simulink model "project1_Jaden"  (R2015b)
settings: Solver=ode45  SolverMode=SingleTasking  StartTime=0.0  StopTime=604800  MaxStep=1  RelTol=1e-6
undefined symbols (not defined in the file or in its folder): plecs, sigbuilder_block
settings Model: Creator=Sam Murray  LastModifiedBy=Sam Murray
settings DataIOCC: SaveFormat=Array
settings OptimizationCC: BlockReduction=off  BooleanDataType=off
settings DebuggingCC: SaveWithParameterizedLinksMsg=none  UnderspecifiedInitializationDetection=Classic  MergeDetectMultiDrivingBlocksExec=none  SignalResolutionControl=TryResolveAllWithWarning  AllowSymbolicDim=on
settings HardwareCC: ProdBitPerPointer=32  ProdLargestAtomicFloat=None  ProdIntDivRoundTo=Undefined  ProdEndianess=Unspecified  ProdWordSize=32  ProdHWDeviceType=32-bit Generic  TargetUnknown=on
settings GRTTargetCC: GeneratePreprocessorConditionals=Disable all
settings ConfigComp: CovMetricSettings=dwe  CovHtmlReporting=off  CovSaveCumulativeToWorkspaceVar=off  CovSaveSingleToWorkspaceVar=off  CovModelRefEnable=Off  CovExternalEMLEnable=on

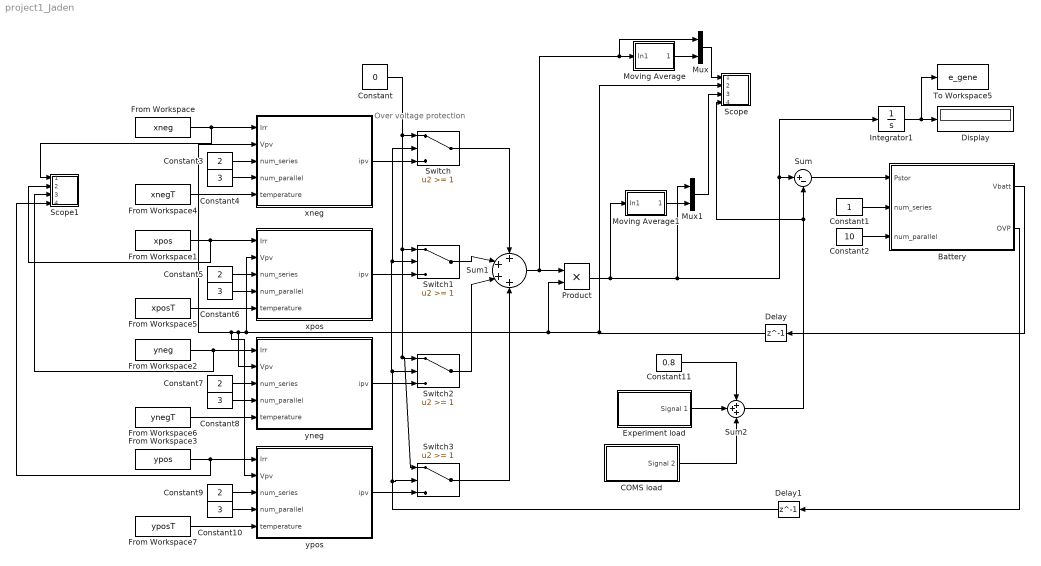
== system project1_Jaden ==
  note: Over voltage protection
  Battery : Subsystem
  COMS load : Subsystem  Tag=STV Subsys  LoadFcn=sigbuilder_block('load');  StartFcn=sigbuilder_block('start');  StopFcn=sigbuilder_block('stop');  ClipboardFcn=sigbuilder_block('clipboard');  mask(Sigbuilder block){}
      mask help: Simulink:masks:SigbuilderBlock_MD
      mask init:
      | if ~strcmp(get_param(bdroot(gcbh),'SimulationStatus'),'stopped') tuvar = sigbuilder_block('maskInit'); end
      settings: CopyFcn=sigbuilder_block('copy');  DeleteFcn=sigbuilder_block('delete');  ModelCloseFcn=sigbuilder_block('modelClose');  PreSaveFcn=sigbuilder_block('preSave');  PauseFcn=sigbuilder_block('pause');  ContinueFcn=sigbuilder_block('continue');  NameChangeFcn=sigbuilder_block('namechange');  OpenFcn=sigbuilder_block('open',[312.75 246 827.25 429 ]);  CloseFcn=sigbuilder_block('close');
      mask Display: plot(0, 0, 100, 100,[2, 2, 32, 32, 2], [68, 8, 8, 68, 68],[32, 2], [38, 38], [32, 19, 2],[53, 60, 44], [32, 17, 17, 2],[16, 16, 31, 31]);txt = getActiveGroup(gcbh);text(2, 100, txt,'verticalAlignment', 'top');
  Constant : Constant  Value=0
  Constant1 : Constant
  Constant{4,6,8,10} (4 alike) : Constant  Value=3
  Constant11 : Constant  Value=0.8
  Constant2 : Constant  Value=10
  Constant{3,5,7,9} (4 alike) : Constant  Value=2
  Delay : Delay  DelayLength=1  InitialCondition=0
  Delay1 : Delay  DelayLength=1  InitialCondition=0
  Display : Display
  Experiment load : Subsystem  Tag=STV Subsys  LoadFcn=sigbuilder_block('load');  StartFcn=sigbuilder_block('start');  StopFcn=sigbuilder_block('stop');  ClipboardFcn=sigbuilder_block('clipboard');  mask(Sigbuilder block){}
      mask help: Simulink:masks:SigbuilderBlock_MD
      mask init:
      | if ~strcmp(get_param(bdroot(gcbh),'SimulationStatus'),'stopped') tuvar = sigbuilder_block('maskInit'); end
      settings: CopyFcn=sigbuilder_block('copy');  DeleteFcn=sigbuilder_block('delete');  ModelCloseFcn=sigbuilder_block('modelClose');  PreSaveFcn=sigbuilder_block('preSave');  PauseFcn=sigbuilder_block('pause');  ContinueFcn=sigbuilder_block('continue');  NameChangeFcn=sigbuilder_block('namechange');  OpenFcn=sigbuilder_block('open',[312.75 246 827.25 429 ]);  CloseFcn=sigbuilder_block('close');
      mask Display: plot(0, 0, 100, 100,[2, 2, 32, 32, 2], [68, 8, 8, 68, 68],[32, 2], [38, 38], [32, 19, 2],[53, 60, 44], [32, 17, 17, 2],[16, 16, 31, 31]);txt = getActiveGroup(gcbh);text(2, 100, txt,'verticalAlignment', 'top');
  From Workspace : FromWorkspace  VariableName=xneg  SampleTime=0
  From Workspace1 : FromWorkspace  VariableName=xpos  SampleTime=0
  From Workspace2 : FromWorkspace  VariableName=yneg  SampleTime=0
  From Workspace3 : FromWorkspace  VariableName=ypos  SampleTime=0
  From Workspace4 : FromWorkspace  VariableName=xnegT  SampleTime=0
  From Workspace5 : FromWorkspace  VariableName=xposT  SampleTime=0
  From Workspace6 : FromWorkspace  VariableName=ynegT  SampleTime=0
  From Workspace7 : FromWorkspace  VariableName=yposT  SampleTime=0
  Integrator1 : Integrator
  Moving Average : Subsystem  Description=Replaced Block  mask(Replaced Block){}
      mask help: This block has been replaced with an empty subsystem because it used functionality that is unavailable in Simulink R2015b.
      mask Display: fprintf('Replaced: %s\n','dspstat3/Moving Average')
  Moving Average1 : Subsystem  Description=Replaced Block  mask(Replaced Block){}
      mask help: This block has been replaced with an empty subsystem because it used functionality that is unavailable in Simulink R2015b.
      mask Display: fprintf('Replaced: %s\n','dspstat3/Moving Average')
  Mux : Mux  Inputs=2
  Mux1 : Mux  Inputs=2
  Product : Product
  Scope : Subsystem  LoadFcn=plecs('sl', 300);  InitFcn=plecs('sl', 314);  StartFcn=plecs('sl', 308);  StopFcn=plecs('sl', 309);  mask{Settings=<binary blob, 1724 chars, not shown>}
      mask init:
      | plecs('sl', 315);
      settings: CopyFcn=plecs('sl', 303);  DeleteFcn=plecs('sl', 305);  UndoDeleteFcn=plecs('sl', 306);  PreSaveFcn=plecs('sl', 311);  NameChangeFcn=plecs('sl', 310);  DestroyFcn=plecs('sl', 307);  OpenFcn=plecs('sl', 302);  ErrorFcn=plerrorfcn
      mask Display: plot([0.1 0.9 0.9 0.1 0.1], [0.9 0.9 0.5 0.5 0.9])
  Scope1 : Subsystem  LoadFcn=plecs('sl', 300);  InitFcn=plecs('sl', 314);  StartFcn=plecs('sl', 308);  StopFcn=plecs('sl', 309);  mask{Settings=<binary blob, 1460 chars, not shown>}
      mask init:
      | plecs('sl', 315);
      settings: CopyFcn=plecs('sl', 303);  DeleteFcn=plecs('sl', 305);  UndoDeleteFcn=plecs('sl', 306);  PreSaveFcn=plecs('sl', 311);  NameChangeFcn=plecs('sl', 310);  DestroyFcn=plecs('sl', 307);  OpenFcn=plecs('sl', 302);  ErrorFcn=plerrorfcn
      mask Display: plot([0.1 0.9 0.9 0.1 0.1], [0.9 0.9 0.5 0.5 0.9])
  Sum : Sum  Inputs=|+-
  Sum1 : Sum  Inputs=++++
  Sum2 : Sum  Inputs=+++
  Switch{,1..3} (4 alike) : Switch  Threshold=1
  To Workspace5 : ToWorkspace  VariableName=e_gene  SaveFormat=Timeseries  SampleTime=-1
  xneg : Subsystem
  xpos : Subsystem
  yneg : Subsystem
  ypos : Subsystem
  wires:
  Constant1/1 -> Battery/2(num_series)
  Constant2/1 -> Battery/3(num_parallel)
  Constant4/1 -> xneg/4(num_parallel)
  Constant3/1 -> xneg/3(num_series)
  Sum/1 -> Battery/1(Pstor)
  From Workspace2/1 -> yneg/1(Irr), Scope1/3(3)
  From Workspace1/1 -> xpos/1(Irr), Scope1/2(2)
  From Workspace3/1 -> ypos/1(Irr), Scope1/4(4)
  Battery/1(Vbatt) -> Delay/1
  Sum1/1 -> Mux/1, Moving Average/1(In1), Product/1
  Product/1 -> Mux1/1, Integrator1/1, Sum/1, Moving Average1/1(In1)
  From Workspace/1 -> Scope1/1(1), xneg/1(Irr)
  Delay/1 -> Scope/2(2), Product/2, xpos/2(Vpv), yneg/2(Vpv), ypos/2(Vpv), xneg/2(Vpv)
  Switch/1 -> Sum1/1
  xneg/1(ipv) -> Switch/3
  Switch1/1 -> Sum1/2
  xpos/1(ipv) -> Switch1/3
  Switch2/1 -> Sum1/3
  yneg/1(ipv) -> Switch2/3
  ypos/1(ipv) -> Switch3/3
  Constant/1 -> Switch3/1, Switch2/1, Switch1/1, Switch/1
  Battery/2(OVP) -> Delay1/1
  Delay1/1 -> Switch3/2, Switch/2, Switch1/2, Switch2/2
  Integrator1/1 -> To Workspace5/1, Display/1
  Sum2/1 -> Scope/4(4), Sum/2
  Constant11/1 -> Sum2/1
  Experiment load/1(Signal 1) -> Sum2/2
  COMS load/1(Signal 2) -> Sum2/3
  Mux/1 -> Scope/1(1)
  Mux1/1 -> Scope/3(3)
  Moving Average1/1(Out1) -> Mux1/2
  Moving Average/1(Out1) -> Mux/2
  Constant5/1 -> xpos/3(num_series)
  Constant6/1 -> xpos/4(num_parallel)
  Constant7/1 -> yneg/3(num_series)
  Constant8/1 -> yneg/4(num_parallel)
  Constant9/1 -> ypos/3(num_series)
  Constant10/1 -> ypos/4(num_parallel)
  From Workspace4/1 -> xneg/5(temperature)
  From Workspace5/1 -> xpos/5(temperature)
  From Workspace6/1 -> yneg/5(temperature)
  From Workspace7/1 -> ypos/5(temperature)
  Switch3/1 -> Sum1/4

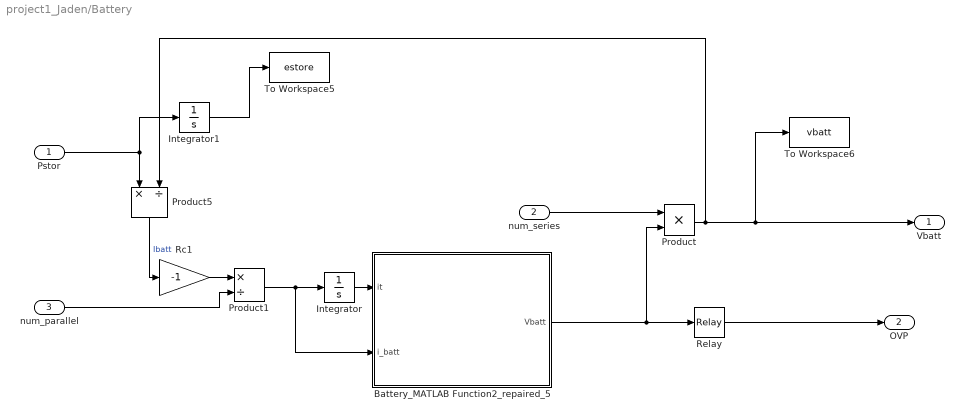
== system project1_Jaden/Battery ==
  Pstor : Inport
  num_series : Inport  Port=2
  num_parallel : Inport  Port=3
  Battery_MATLAB Function2_repaired_5 : MATLAB Function
  Integrator : Integrator  InitialCondition=4680
  Integrator1 : Integrator
  Product : Product
  Product1 : Product  Inputs=*/
  Product5 : Product  Inputs=*/  OutMin=[0]
  Rc1 : Gain  Gain=-1
  Relay : Relay  OnSwitchValue=4.2  OffSwitchValue=4.18
  To Workspace5 : ToWorkspace  VariableName=estore  SaveFormat=Timeseries  SampleTime=-1
  To Workspace6 : ToWorkspace  VariableName=vbatt  SaveFormat=Timeseries  SampleTime=-1
  Vbatt : Outport
  OVP : Outport  Port=2
  wires:
  Product/1 -> Product5/2, Vbatt/1, To Workspace6/1
  Battery_MATLAB Function2_repaired_5/1(Vbatt) -> Product/2, Relay/1
  num_series/1 -> Product/1
  num_parallel/1 -> Product1/2
  Product1/1 -> Battery_MATLAB Function2_repaired_5/2(i_batt), Integrator/1
  Integrator/1 -> Battery_MATLAB Function2_repaired_5/1(it)
  Relay/1 -> OVP/1
  Rc1/1 -> Product1/1
  Pstor/1 -> Product5/1, Integrator1/1
  Product5/1 -> Rc1/1  "Ibatt"
  Integrator1/1 -> To Workspace5/1

== system project1_Jaden/COMS load ==
  Demux : Demux  Tag=STV Demux  Outputs=1
  FromWs : FromWorkspace  Tag=STV FromWs  VariableName=tuvar  SampleTime=0
      SigBuilderData=|
      | common.afterFinalStr = 'Extrapolate'
      | common.sampleTime = 0
      | dataSet.timeRange = [0 604800]
      | dataSet.name = 'Group 1'
      | sbobj.Groups.Name = 'Group 1'
      | sbobj.Groups.Signals.Name = 'Signal 2'
      | sbobj.Groups.Signals.XData = [0 60 60 14400 14400 14460 14460 28800 28800 28860 28860 43200 43200 43260 43260 57600 57600 57660 57660 72000 72000 72060 72060 86400 86400 86460 86460 100800 100800 100860 100860 115200 115200 115260 115260 129600 129600 129660 129660 144000 144000 144060 144060 158400 158400 158460 158460 172800 172800 172860 172860 187200 187200 187260 187260 201600 201600 201660 201660 216000 216000 216060 216060 230400 230400 230460 230460 244800 244800 244860 244860 259200 259200 259260 259260 273600 273600 273660 273660 288000 288000 288060 288060 302400 302400 302460 302460 316800 316800 316860 316860 331200 331200 331260 331260 345600 345600 345660 345660 360000 360000 360060 360060 374400 374400 374460 374460 388800 388800 388860 388860 403200 403200 403260 403260 417600 417600 417660 417660 432000 432000 432060 432060 446400 446400 446460 446460 460800 460800 460860 460860 475200 475200 475260 475260 489600 489600 489660 489660 504000 504000 504060 504060 518400 518400 518460 518460 532800 532800 532860 532860 547200 547200 547260 547260 561600 561600 561660 561660 576000 576000 576060 576060 590400 590400 590460 590460 604800]
      | sbobj.Groups.Signals.YData = [5 5 0 0 5 5 0 0 5 5 0 0 5 5 0 0 5 5 0 0 5 5 0 0 5 5 0 0 5 5 0 0 5 5 0 0 5 5 0 0 5 5 0 0 5 5 0 0 5 5 0 0 5 5 0 0 5 5 0 0 5 5 0 0 5 5 0 0 5 5 0 0 5 5 0 0 5 5 0 0 5 5 0 0 5 5 0 0 5 5 0 0 5 5 0 0 5 5 0 0 5 5 0 0 5 5 0 0 5 5 0 0 5 5 0 0 5 5 0 0 5 5 0 0 5 5 0 0 5 5 0 0 5 5 0 0 5 5 0 0 5 5 0 0 5 5 0 0 5 5 0 0 5 5 0 0 5 5 0 0 5 5 0 0 5 5 0 0]
      | sbobj.Groups.TimeRange = [0 604800]
  Signal 2 : Outport  Tag=STV Outport
  wires:
  FromWs/1 -> Demux/1
  Demux/1 -> Signal 2/1

== system project1_Jaden/Experiment load ==
  Demux : Demux  Tag=STV Demux  Outputs=1
  FromWs : FromWorkspace  Tag=STV FromWs  VariableName=tuvar  SampleTime=0
      SigBuilderData=|
      | common.afterFinalStr = 'Extrapolate'
      | common.sampleTime = 0
      | dataSet.timeRange = [0 604800]
      | dataSet.name = 'Group 1'
      | sbobj.Groups.Name = 'Group 1'
      | sbobj.Groups.Signals.Name = 'Signal 1'
      | sbobj.Groups.Signals.XData = [0 196000 200000 200000 373000 373000 604800]
      | sbobj.Groups.Signals.YData = [0 0 2.5 3.75 3.75 0 0]
      | sbobj.Groups.TimeRange = [0 604800]
  Signal 1 : Outport  Tag=STV Outport
  wires:
  FromWs/1 -> Demux/1
  Demux/1 -> Signal 1/1

== system project1_Jaden/Moving Average ==
  In1 : Inport
  Ground1 : Ground
  Terminator1 : Terminator
  Out1 : Outport
  wires:
  Ground1/1 -> Out1/1
  In1/1 -> Terminator1/1

== system project1_Jaden/Moving Average1 ==
  In1 : Inport
  Ground1 : Ground
  Terminator1 : Terminator
  Out1 : Outport
  wires:
  Ground1/1 -> Out1/1
  In1/1 -> Terminator1/1

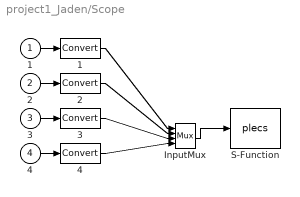
== system project1_Jaden/Scope ==
  1 : Inport
  2 : Inport  Port=2
  3 : Inport  Port=3
  4 : Inport  Port=4
  " 1 " : DataTypeConversion  SaturateOnIntegerOverflow=on  RndMeth=Zero
  " 2 " : DataTypeConversion  SaturateOnIntegerOverflow=on  RndMeth=Zero
  " 3 " : DataTypeConversion  SaturateOnIntegerOverflow=on  RndMeth=Zero
  " 4 " : DataTypeConversion  SaturateOnIntegerOverflow=on  RndMeth=Zero
  " InputMux " : Mux
  " S-Function " : S-Function  FunctionName=plecs  SFunctionDeploymentMode=off  EnableBusSupport=off
  wires:
  " InputMux "/1 -> " S-Function "/1
  1/1 -> " 1 "/1
  " 1 "/1 -> " InputMux "/1
  2/1 -> " 2 "/1
  " 2 "/1 -> " InputMux "/2
  3/1 -> " 3 "/1
  " 3 "/1 -> " InputMux "/3
  4/1 -> " 4 "/1
  " 4 "/1 -> " InputMux "/4

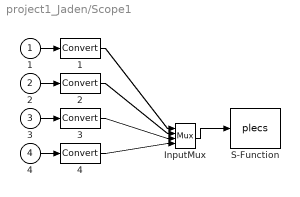
== system project1_Jaden/Scope1 ==
  1 : Inport
  2 : Inport  Port=2
  3 : Inport  Port=3
  4 : Inport  Port=4
  " 1 " : DataTypeConversion  SaturateOnIntegerOverflow=on  RndMeth=Zero
  " 2 " : DataTypeConversion  SaturateOnIntegerOverflow=on  RndMeth=Zero
  " 3 " : DataTypeConversion  SaturateOnIntegerOverflow=on  RndMeth=Zero
  " 4 " : DataTypeConversion  SaturateOnIntegerOverflow=on  RndMeth=Zero
  " InputMux " : Mux
  " S-Function " : S-Function  FunctionName=plecs  SFunctionDeploymentMode=off  EnableBusSupport=off
  wires:
  " InputMux "/1 -> " S-Function "/1
  1/1 -> " 1 "/1
  " 1 "/1 -> " InputMux "/1
  2/1 -> " 2 "/1
  " 2 "/1 -> " InputMux "/2
  3/1 -> " 3 "/1
  " 3 "/1 -> " InputMux "/3
  4/1 -> " 4 "/1
  " 4 "/1 -> " InputMux "/4

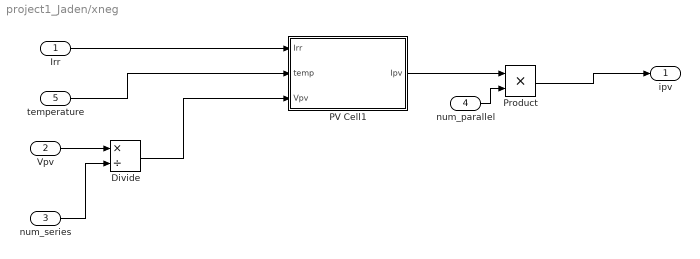
== system project1_Jaden/xneg ==
  Irr : Inport
  Vpv : Inport  Port=2
  num_series : Inport  Port=3
  num_parallel : Inport  Port=4
  temperature : Inport  Port=5
  Divide : Product  Inputs=*/
  PV Cell1 : Subsystem
  Product : Product
  ipv : Outport
  wires:
  Irr/1 -> PV Cell1/1(Irr)
  Vpv/1 -> Divide/1
  num_series/1 -> Divide/2
  Divide/1 -> PV Cell1/3(Vpv)
  PV Cell1/1(Ipv) -> Product/1
  Product/1 -> ipv/1
  num_parallel/1 -> Product/2
  temperature/1 -> PV Cell1/2(temp)

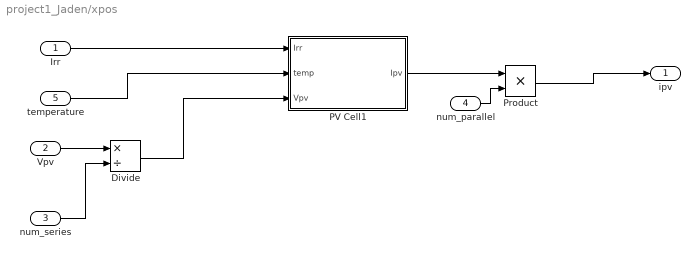
== system project1_Jaden/xpos ==
  Irr : Inport
  Vpv : Inport  Port=2
  num_series : Inport  Port=3
  num_parallel : Inport  Port=4
  temperature : Inport  Port=5
  Divide : Product  Inputs=*/
  PV Cell1 : Subsystem
  Product : Product
  ipv : Outport
  wires:
  Irr/1 -> PV Cell1/1(Irr)
  Vpv/1 -> Divide/1
  num_series/1 -> Divide/2
  Divide/1 -> PV Cell1/3(Vpv)
  PV Cell1/1(Ipv) -> Product/1
  Product/1 -> ipv/1
  num_parallel/1 -> Product/2
  temperature/1 -> PV Cell1/2(temp)

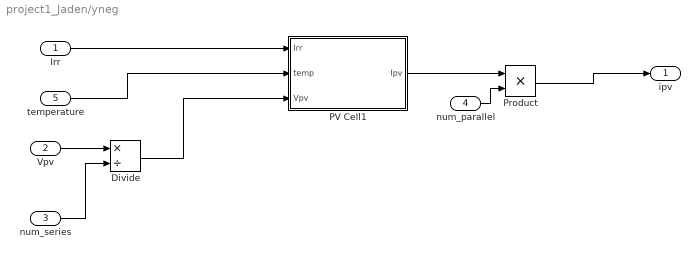
== system project1_Jaden/yneg ==
  Irr : Inport
  Vpv : Inport  Port=2
  num_series : Inport  Port=3
  num_parallel : Inport  Port=4
  temperature : Inport  Port=5
  Divide : Product  Inputs=*/
  PV Cell1 : Subsystem
  Product : Product
  ipv : Outport
  wires:
  Irr/1 -> PV Cell1/1(Irr)
  Vpv/1 -> Divide/1
  num_series/1 -> Divide/2
  Divide/1 -> PV Cell1/3(Vpv)
  PV Cell1/1(Ipv) -> Product/1
  Product/1 -> ipv/1
  num_parallel/1 -> Product/2
  temperature/1 -> PV Cell1/2(temp)

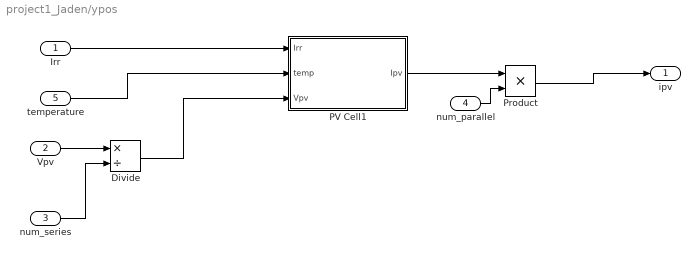
== system project1_Jaden/ypos ==
  Irr : Inport
  Vpv : Inport  Port=2
  num_series : Inport  Port=3
  num_parallel : Inport  Port=4
  temperature : Inport  Port=5
  Divide : Product  Inputs=*/
  PV Cell1 : Subsystem
  Product : Product
  ipv : Outport
  wires:
  Irr/1 -> PV Cell1/1(Irr)
  Vpv/1 -> Divide/1
  num_series/1 -> Divide/2
  Divide/1 -> PV Cell1/3(Vpv)
  PV Cell1/1(Ipv) -> Product/1
  Product/1 -> ipv/1
  num_parallel/1 -> Product/2
  temperature/1 -> PV Cell1/2(temp)

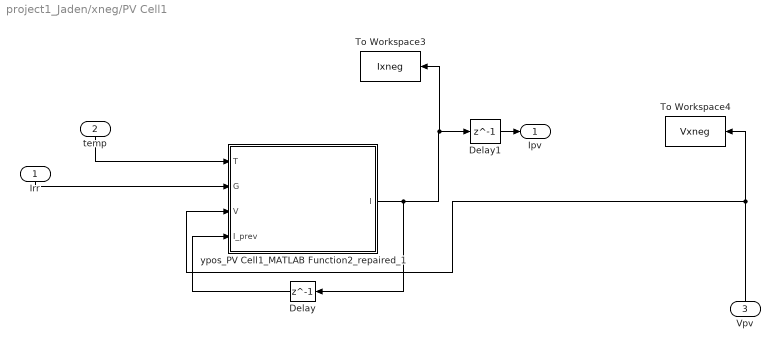
== system project1_Jaden/xneg/PV Cell1 ==
  Irr : Inport
  temp : Inport  Port=2
  Vpv : Inport  Port=3
  Delay : Delay  DelayLength=1  InitialCondition=0
  Delay1 : Delay  DelayLength=1  InitialCondition=0
  To Workspace3 : ToWorkspace  VariableName=Ixneg  SaveFormat=Timeseries  SampleTime=-1
  To Workspace4 : ToWorkspace  VariableName=Vxneg  SaveFormat=Timeseries  SampleTime=-1
  ypos_PV Cell1_MATLAB Function2_repaired_1 : MATLAB Function
  Ipv : Outport
  wires:
  Irr/1 -> ypos_PV Cell1_MATLAB Function2_repaired_1/2(G)
  temp/1 -> ypos_PV Cell1_MATLAB Function2_repaired_1/1(T)
  Delay/1 -> ypos_PV Cell1_MATLAB Function2_repaired_1/4(I_prev)
  Vpv/1 -> ypos_PV Cell1_MATLAB Function2_repaired_1/3(V), To Workspace4/1
  ypos_PV Cell1_MATLAB Function2_repaired_1/1(I) -> To Workspace3/1, Delay1/1, Delay/1
  Delay1/1 -> Ipv/1

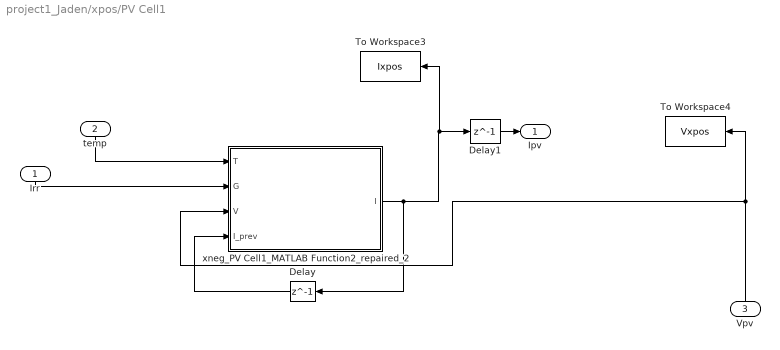
== system project1_Jaden/xpos/PV Cell1 ==
  Irr : Inport
  temp : Inport  Port=2
  Vpv : Inport  Port=3
  Delay : Delay  DelayLength=1  InitialCondition=0
  Delay1 : Delay  DelayLength=1  InitialCondition=0
  To Workspace3 : ToWorkspace  VariableName=Ixpos  SaveFormat=Timeseries  SampleTime=-1
  To Workspace4 : ToWorkspace  VariableName=Vxpos  SaveFormat=Timeseries  SampleTime=-1
  xneg_PV Cell1_MATLAB Function2_repaired_2 : MATLAB Function
  Ipv : Outport
  wires:
  Irr/1 -> xneg_PV Cell1_MATLAB Function2_repaired_2/2(G)
  temp/1 -> xneg_PV Cell1_MATLAB Function2_repaired_2/1(T)
  Delay/1 -> xneg_PV Cell1_MATLAB Function2_repaired_2/4(I_prev)
  Vpv/1 -> xneg_PV Cell1_MATLAB Function2_repaired_2/3(V), To Workspace4/1
  xneg_PV Cell1_MATLAB Function2_repaired_2/1(I) -> To Workspace3/1, Delay1/1, Delay/1
  Delay1/1 -> Ipv/1

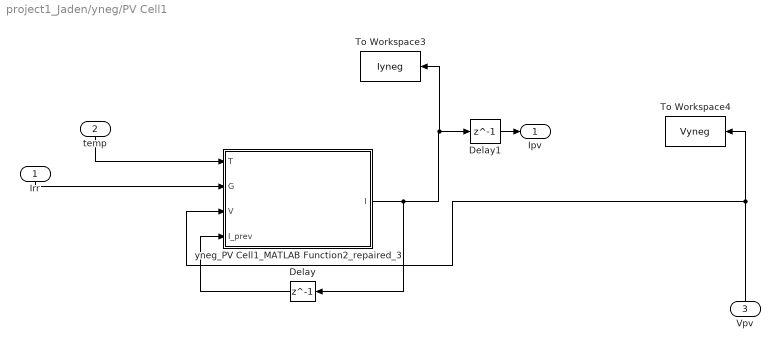
== system project1_Jaden/yneg/PV Cell1 ==
  Irr : Inport
  temp : Inport  Port=2
  Vpv : Inport  Port=3
  Delay : Delay  DelayLength=1  InitialCondition=0
  Delay1 : Delay  DelayLength=1  InitialCondition=0
  To Workspace3 : ToWorkspace  VariableName=Iyneg  SaveFormat=Timeseries  SampleTime=-1
  To Workspace4 : ToWorkspace  VariableName=Vyneg  SaveFormat=Timeseries  SampleTime=-1
  yneg_PV Cell1_MATLAB Function2_repaired_3 : MATLAB Function
  Ipv : Outport
  wires:
  Irr/1 -> yneg_PV Cell1_MATLAB Function2_repaired_3/2(G)
  temp/1 -> yneg_PV Cell1_MATLAB Function2_repaired_3/1(T)
  Delay/1 -> yneg_PV Cell1_MATLAB Function2_repaired_3/4(I_prev)
  Vpv/1 -> yneg_PV Cell1_MATLAB Function2_repaired_3/3(V), To Workspace4/1
  yneg_PV Cell1_MATLAB Function2_repaired_3/1(I) -> To Workspace3/1, Delay1/1, Delay/1
  Delay1/1 -> Ipv/1

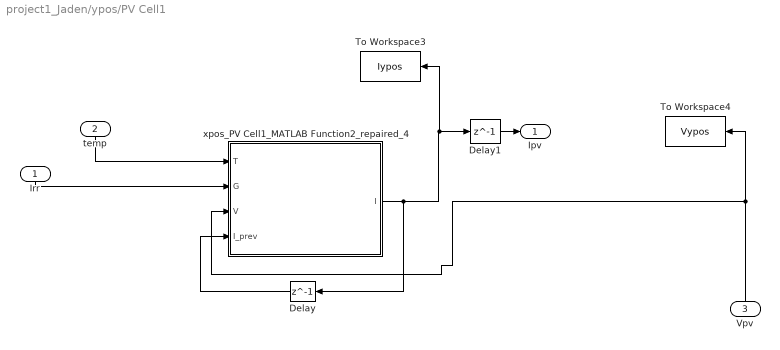
== system project1_Jaden/ypos/PV Cell1 ==
  Irr : Inport
  temp : Inport  Port=2
  Vpv : Inport  Port=3
  Delay : Delay  DelayLength=1  InitialCondition=0
  Delay1 : Delay  DelayLength=1  InitialCondition=0
  To Workspace3 : ToWorkspace  VariableName=Iypos  SaveFormat=Timeseries  SampleTime=-1
  To Workspace4 : ToWorkspace  VariableName=Vypos  SaveFormat=Timeseries  SampleTime=-1
  xpos_PV Cell1_MATLAB Function2_repaired_4 : MATLAB Function
  Ipv : Outport
  wires:
  Irr/1 -> xpos_PV Cell1_MATLAB Function2_repaired_4/2(G)
  temp/1 -> xpos_PV Cell1_MATLAB Function2_repaired_4/1(T)
  Delay/1 -> xpos_PV Cell1_MATLAB Function2_repaired_4/4(I_prev)
  Vpv/1 -> xpos_PV Cell1_MATLAB Function2_repaired_4/3(V), To Workspace4/1
  xpos_PV Cell1_MATLAB Function2_repaired_4/1(I) -> To Workspace3/1, Delay1/1, Delay/1
  Delay1/1 -> Ipv/1

== matlab function project1_Jaden/Battery/Battery_MATLAB Function2_repaired_5 ==
  data: it input; Vbatt output; i_batt input
function Vbatt = battery_eqn(it, i_batt)
% Function that will model the lithium ion battery 

%E = 3.6; % No load voltage (V)
E0 = 3.6;%3.7348; % Battery constant voltage (V)
K = 0.01;%0.00876; %polarisation voltage (V)
Q = 8100; % or 2.87Ah;  % battey capacity (As)
A = 0.7; %0.468; %exponential zone amplitude (V)
B = 0.0003; %3.5294; %exponential zone time constant inverse (Ah)^-1
R = 0.09; % internal resistance (Ohms)

E = E0 - K*(Q/(Q-it)) + A*exp(-B*it); 
Vbatt = E - i_batt*R;
end

== matlab function project1_Jaden/xpos/PV Cell1/xneg_PV Cell1_MATLAB Function2_repaired_2 ==
  data: T input; I output; G input; V input; I_prev input
function I = pv_module(T,G,V, I_prev)
    %Code to model the output of a solar cell 

    %Intrinsic Parameters 
    Gn = 1395; % In W/m^3
    delta_T = T - (25+273); %in degK
    Iscn = 0.45387; % in amps
    Vocn = 2.660; % in volts
    Ns = 1;
    Ki = 0; %0.000141 ;  % Thermal coefficient of Isc (in A/degC)
    Kv = 0; %-0.0059 ;  % thermal coefficient of Voc (in A/degC)
    I_pvn = 0.45387; % in amps
    a = 2.8; %diode ideality constant (between 1 and 1.5)
    q = 1.60217646e-19;
    k = 1.3806503e-23;
    Vt = (Ns*k*(T))/q; % thermal voltage of Ns series connected cells

    % Parameters that I have to tune
    Rs = 0.17; %0.235; %0.005649;
    Rp = 560; %560;

    % Calculating the different solar currents 
    I_pv = (I_pvn + Ki*delta_T)*(G/Gn);

    I_o = (Iscn + Ki*delta_T) / (exp((Vocn + Kv*delta_T)/(a*Vt)) - 1); 

    I_dio = I_o*( exp((V + Rs*I_prev)/(Vt*a)) -1 );

    I_res_loss = (V + Rs*I_prev) / Rp;

    I = I_pv - I_res_loss - I_dio;
end

== matlab function project1_Jaden/ypos/PV Cell1/xpos_PV Cell1_MATLAB Function2_repaired_4 ==
  data: T input; I output; G input; V input; I_prev input
function I = pv_module(T,G,V, I_prev)
    %Code to model the output of a solar cell 

    %Intrinsic Parameters 
    Gn = 1395; % In W/m^3
    delta_T = T - (25+273); %in degK
    Iscn = 0.45387; % in amps
    Vocn = 2.660; % in volts
    Ns = 1;
    Ki = 0; %0.000141 ;  % Thermal coefficient of Isc (in A/degC)
    Kv = 0; %-0.0059 ;  % thermal coefficient of Voc (in A/degC)
    I_pvn = 0.45387; % in amps
    a = 2.8; %diode ideality constant (between 1 and 1.5)
    q = 1.60217646e-19;
    k = 1.3806503e-23;
    Vt = (Ns*k*(T))/q; % thermal voltage of Ns series connected cells

    % Parameters that I have to tune
    Rs = 0.17; %0.235; %0.005649;
    Rp = 560; %560;

    % Calculating the different solar currents 
    I_pv = (I_pvn + Ki*delta_T)*(G/Gn);

    I_o = (Iscn + Ki*delta_T) / (exp((Vocn + Kv*delta_T)/(a*Vt)) - 1); 

    I_dio = I_o*( exp((V + Rs*I_prev)/(Vt*a)) -1 );

    I_res_loss = (V + Rs*I_prev) / Rp;

    I = I_pv - I_res_loss - I_dio;
end

== matlab function project1_Jaden/yneg/PV Cell1/yneg_PV Cell1_MATLAB Function2_repaired_3 ==
  data: T input; I output; G input; V input; I_prev input
function I = pv_module(T,G,V, I_prev)
    %Code to model the output of a solar cell 

    %Intrinsic Parameters 
    Gn = 1395; % In W/m^3
    delta_T = T - (25+273); %in degK
    Iscn = 0.45387; % in amps
    Vocn = 2.660; % in volts
    Ns = 1;
    Ki = 0; %0.000141 ;  % Thermal coefficient of Isc (in A/degC)
    Kv = 0; %-0.0059 ;  % thermal coefficient of Voc (in A/degC)
    I_pvn = 0.45387; % in amps
    a = 2.8; %diode ideality constant (between 1 and 1.5)
    q = 1.60217646e-19;
    k = 1.3806503e-23;
    Vt = (Ns*k*(T))/q; % thermal voltage of Ns series connected cells

    % Parameters that I have to tune
    Rs = 0.17; %0.235; %0.005649;
    Rp = 560; %560;

    % Calculating the different solar currents 
    I_pv = (I_pvn + Ki*delta_T)*(G/Gn);

    I_o = (Iscn + Ki*delta_T) / (exp((Vocn + Kv*delta_T)/(a*Vt)) - 1); 

    I_dio = I_o*( exp((V + Rs*I_prev)/(Vt*a)) -1 );

    I_res_loss = (V + Rs*I_prev) / Rp;

    I = I_pv - I_res_loss - I_dio;
end

== matlab function project1_Jaden/xneg/PV Cell1/ypos_PV Cell1_MATLAB Function2_repaired_1 ==
  data: T input; I output; G input; V input; I_prev input
function I = pv_module(T,G,V, I_prev)
    %Code to model the output of a solar cell 

    %Intrinsic Parameters 
    Gn = 1395; % In W/m^3
    delta_T = T - (25+273); %in degC
    Iscn = 0.45387; % in amps
    Vocn = 2.660; % in volts
    Ns = 1;
    Ki = 0; %0.000141 ;  % Thermal coefficient of Isc (in A/degC)
    Kv = 0; %-0.0059 ;  % thermal coefficient of Voc (in A/degC)
    I_pvn = 0.45387; % in amps
    a = 2.8; %diode ideality constant (between 1 and 1.5)
    q = 1.60217646e-19;
    k = 1.3806503e-23;
    Vt = (Ns*k*(T))/q; % thermal voltage of Ns series connected cells

    % Parameters that I have to tune
    Rs = 0.17; %0.235; %0.005649;
    Rp = 560; %560;

    % Calculating the different solar currents 
    I_pv = (I_pvn + Ki*delta_T)*(G/Gn);

    I_o = (Iscn + Ki*delta_T) / (exp((Vocn + Kv*delta_T)/(a*Vt)) - 1); 

    I_dio = I_o*( exp((V + Rs*I_prev)/(Vt*a)) -1 );

    I_res_loss = (V + Rs*I_prev) / Rp;

    I = I_pv - I_res_loss - I_dio;
end
